simulink model "SystemControl"  (R2019b)
settings: Solver=VariableStepAuto  StartTime=0.0  StopTime=T_sim  RelTol=1e-3
values from neighbouring files (symbols this model uses):
  d_tank = 0.07    [FullSystem.m]    (also in SystemControl_script.m)
  k_m_t = 23.8e-3    (= 0.0238)    [FullSystem.m]    (also in SystemControl_script.m)
  R_load = 1e3    (= 1000)    [FullSystem.m]    (also in SystemControl_script.m)
  T_sim = 5    [FullSystem.m]    (also in SystemControl_script.m = 10; model_1.m = 24)
undefined symbols (not defined in the file or in its folder): columns, DiscIntNeverNeededParam, I_LED_max, V_electrolyzer, V_network
libraries: simulink x5
settings Model: Creator=thequ  LastModifiedBy=thequ

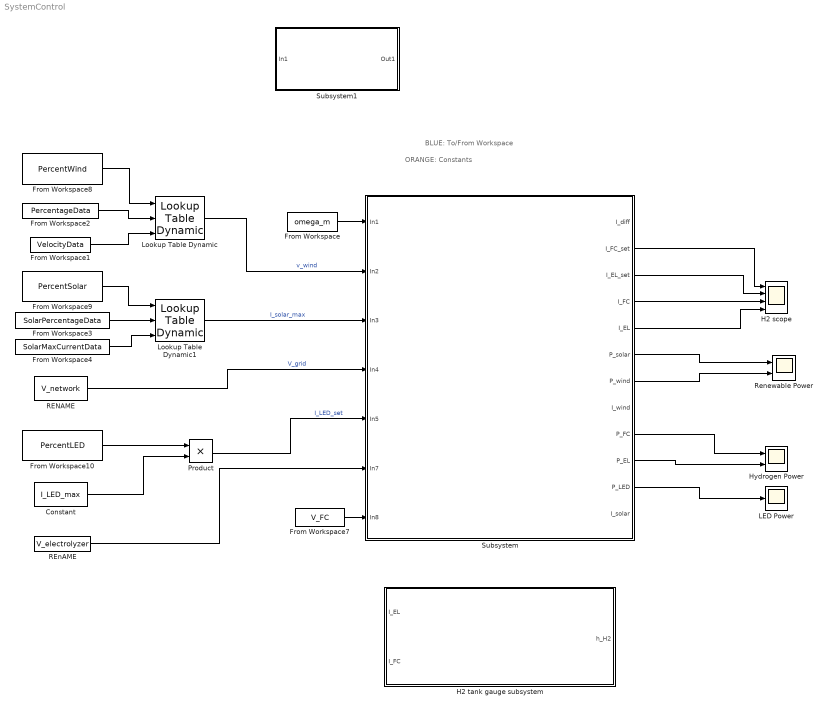
== system SystemControl ==
  note: ORANGE: Constants
  note: BLUE: To/From Workspace
  Constant : Constant  Value=I_LED_max
  From Workspace : FromWorkspace  VariableName=omega_m  SampleTime=T_sim/(columns-1)  Interpolate=off  OutputAfterFinalValue=Holding final value
  From Workspace1 : FromWorkspace  VariableName=VelocityData  SampleTime=0
  From Workspace10 : FromWorkspace  VariableName=PercentLED  SampleTime=0
  From Workspace2 : FromWorkspace  VariableName=PercentageData  SampleTime=0
  From Workspace3 : FromWorkspace  VariableName=SolarPercentageData  SampleTime=0
  From Workspace4 : FromWorkspace  VariableName=SolarMaxCurrentData  SampleTime=0
  From Workspace7 : FromWorkspace  VariableName=V_FC  SampleTime=T_sim/(columns-1)  Interpolate=off  OutputAfterFinalValue=Holding final value
  From Workspace8 : FromWorkspace  VariableName=PercentWind  SampleTime=0
  From Workspace9 : FromWorkspace  VariableName=PercentSolar  SampleTime=0
  H2 scope : Scope  NumInputPorts=4
  H2 tank gauge subsystem : Subsystem
  Hydrogen Power : Scope  NumInputPorts=2
  LED Power : Scope
  Lookup Table Dynamic : simulink/Lookup Tables/Lookup Table Dynamic  LookUpMeth=Interpolation-Use End Values  OutDataType=fixdt('double')  OutScaling=[]  OutputDataTypeScalingMode=Specify via dialog  OutDataTypeStr=double  DoSatur=off
      settings: SourceProductName=Simulink
  Lookup Table Dynamic1 : simulink/Lookup Tables/Lookup Table Dynamic  LookUpMeth=Interpolation-Use End Values  OutDataType=fixdt('double')  OutScaling=[]  OutputDataTypeScalingMode=Specify via dialog  OutDataTypeStr=double  DoSatur=off
      settings: SourceProductName=Simulink
  Product : Product
  RENAME : Constant  Value=V_network
  REnAME : Constant  Value=V_electrolyzer
  Renewable Power : Scope  NumInputPorts=2
  Subsystem : Subsystem
  Subsystem1 : Subsystem
  wires:
  From Workspace/1 -> Subsystem/1(In1)
  Lookup Table Dynamic/1 -> Subsystem/2(In2)  "v_wind"
  Lookup Table Dynamic1/1 -> Subsystem/3(In3)  "I_solar_max"
  RENAME/1 -> Subsystem/4(In4)  "V_grid"
  Product/1 -> Subsystem/5(In5)  "I_LED_set"
  REnAME/1 -> Subsystem/6(In7)
  From Workspace7/1 -> Subsystem/7(In8)
  Subsystem/2(I_FC_set) -> H2 scope/1
  Subsystem/3(I_EL_set) -> H2 scope/2
  Subsystem/6(P_solar) -> Renewable Power/1
  Subsystem/7(P_wind) -> Renewable Power/2
  Subsystem/9(P_FC) -> Hydrogen Power/1
  Subsystem/10(P_EL) -> Hydrogen Power/2
  Subsystem/11(P_LED) -> LED Power/1
  Constant/1 -> Product/2
  From Workspace10/1 -> Product/1
  From Workspace9/1 -> Lookup Table Dynamic1/1
  Subsystem/4(I_FC) -> H2 scope/3
  Subsystem/5(I_EL) -> H2 scope/4
  From Workspace1/1 -> Lookup Table Dynamic/3
  From Workspace2/1 -> Lookup Table Dynamic/2
  From Workspace8/1 -> Lookup Table Dynamic/1
  From Workspace3/1 -> Lookup Table Dynamic1/2
  From Workspace4/1 -> Lookup Table Dynamic1/3

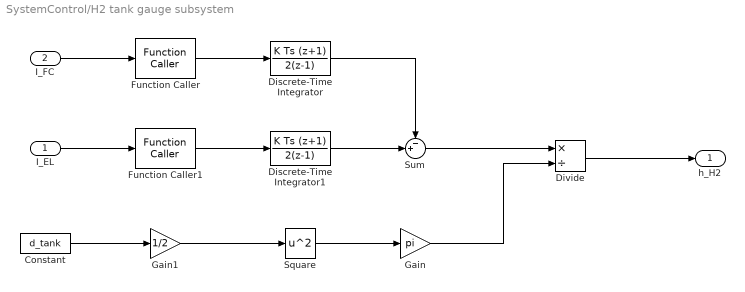
== system SystemControl/H2 tank gauge subsystem ==
  I_EL : Inport
  I_FC : Inport  Port=2
  Constant : Constant  Value=d_tank
  Discrete-Time Integrator : DiscreteIntegrator  IntegratorMethod=Integration: Trapezoidal  SampleTime=-1  ICPrevOutput=DiscIntNeverNeededParam  ICPrevScaledInput=DiscIntNeverNeededParam
  Discrete-Time Integrator1 : DiscreteIntegrator  IntegratorMethod=Integration: Trapezoidal  SampleTime=-1  ICPrevOutput=DiscIntNeverNeededParam  ICPrevScaledInput=DiscIntNeverNeededParam
  Divide : Product  Inputs=*/
  Function Caller : FunctionCaller  FunctionPrototype=y = f(u)  InputArgumentSpecifications=<Enter example>  OutputArgumentSpecifications=<Enter example>
  Function Caller1 : FunctionCaller  FunctionPrototype=y = f(u)  InputArgumentSpecifications=<Enter example>  OutputArgumentSpecifications=<Enter example>
  Gain : Gain  Gain=pi
  Gain1 : Gain  Gain=1/2
  Square : Math  Operator=square  SignedPower=off  SaturateOnIntegerOverflow=on
  Sum : Sum  Inputs=-+|
  h_H2 : Outport
  wires:
  I_FC/1 -> Function Caller/1
  I_EL/1 -> Function Caller1/1
  Function Caller/1 -> Discrete-Time Integrator/1
  Function Caller1/1 -> Discrete-Time Integrator1/1
  Constant/1 -> Gain1/1
  Discrete-Time Integrator1/1 -> Sum/2
  Discrete-Time Integrator/1 -> Sum/1
  Gain1/1 -> Square/1
  Square/1 -> Gain/1
  Gain/1 -> Divide/2
  Sum/1 -> Divide/1
  Divide/1 -> h_H2/1

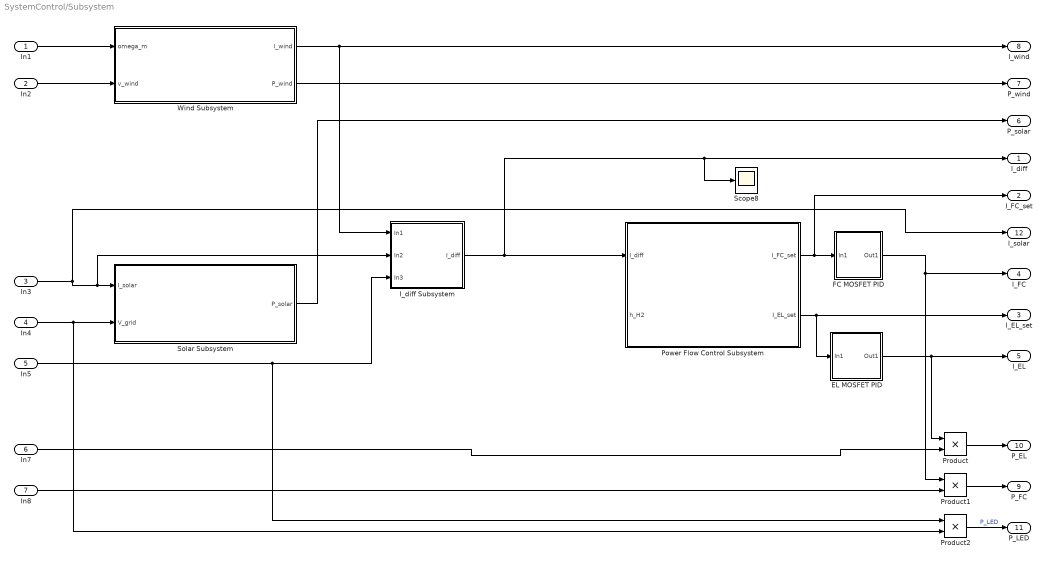
== system SystemControl/Subsystem ==
  In1 : Inport
  In2 : Inport  Port=2
  In3 : Inport  Port=3
  In4 : Inport  Port=4
  In5 : Inport  Port=5
  In7 : Inport  Port=6
  In8 : Inport  Port=7
  EL MOSFET PID : Subsystem
  FC MOSFET PID : Subsystem
  I_diff Subsystem : Subsystem
  Power Flow Control Subsystem : Subsystem
  Product : Product
  Product1 : Product
  Product2 : Product
  Scope8 : Scope
  Solar Subsystem : Subsystem
  "Wind Subsystem " : Subsystem
  I_diff : Outport
  I_FC_set : Outport  Port=2
  I_EL_set : Outport  Port=3
  I_FC : Outport  Port=4
  I_EL : Outport  Port=5
  P_solar : Outport  Port=6
  P_wind : Outport  Port=7
  I_wind : Outport  Port=8
  P_FC : Outport  Port=9
  P_EL : Outport  Port=10
  P_LED : Outport  Port=11
  I_solar : Outport  Port=12
  wires:
  Product2/1 -> P_LED/1  "P_LED"
  I_diff Subsystem/1(I_diff) -> I_diff/1, Scope8/1, Power Flow Control Subsystem/1(I_diff)
  In4/1 -> Product2/2, Solar Subsystem/2(V_grid)
  Power Flow Control Subsystem/2(I_EL_set) -> I_EL_set/1, EL MOSFET PID/1(In1)
  Power Flow Control Subsystem/1(I_FC_set) -> I_FC_set/1, FC MOSFET PID/1(In1)
  EL MOSFET PID/1(Out1) -> I_EL/1, Product/1
  FC MOSFET PID/1(Out1) -> I_FC/1, Product1/1
  In3/1 -> I_diff Subsystem/2(In2), Solar Subsystem/1(I_solar), I_solar/1
  "Wind Subsystem "/2("P_wind ") -> P_wind/1
  "Wind Subsystem "/1("I_wind ") -> I_diff Subsystem/1(In1), I_wind/1
  In5/1 -> Product2/1, I_diff Subsystem/3(In3)
  Product/1 -> P_EL/1
  In1/1 -> "Wind Subsystem "/1(omega_m)
  Product1/1 -> P_FC/1
  Solar Subsystem/1(P_solar) -> P_solar/1
  In2/1 -> "Wind Subsystem "/2("v_wind ")
  In8/1 -> Product1/2
  In7/1 -> Product/2

== system SystemControl/Subsystem1 ==
  In1 : Inport
  Out1 : Outport
  wires:
  In1/1 -> Out1/1

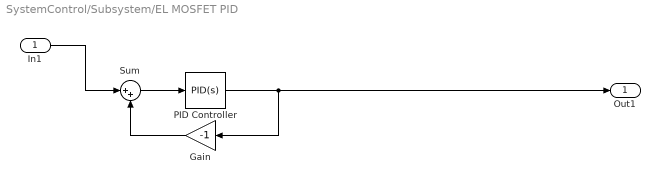
== system SystemControl/Subsystem/EL MOSFET PID ==
  In1 : Inport
  Gain : Gain  Gain=-1
  PID Controller : simulink/Continuous/PID Controller  Controller=PID  Form=Parallel  TimeDomain=Continuous-time  SampleTime=-1  IntegratorMethod=Forward Euler  FilterMethod=Forward Euler  ControllerParametersSource=internal  P=6  I=1  D=0  UseFilter=on  N=100  TunerSelectOption=Transfer Function Based (PID Tuner App)  InitialConditionSource=internal  InitialConditionForIntegrator=0  InitialConditionForFilter=0  DifferentiatorICPrevScaledInput=0  ExternalReset=none  TrackingMode=off  Kt=1  LimitOutput=off  UpperSaturationLimit=inf  LowerSaturationLimit=-inf  LinearizeAsGain=on  AntiWindupMode=none  Kb=1  POutMin=[]  POutMax=[]  IOutMin=[]  IOutMax=[]  DOutMin=[]  DOutMax=[]  NOutMin=[]  NOutMax=[]  SumOutMin=[]  SumOutMax=[]  SaturationOutMin=[]  SaturationOutMax=[]  PParamMin=[]  PParamMax=[]  IParamMin=[]  IParamMax=[]  DParamMin=[]  DParamMax=[]  NParamMin=[]  NParamMax=[]  KbParamMin=[]  KbParamMax=[]  KtParamMin=[]  KtParamMax=[]  KbOutMin=[]  KbOutMax=[]  KtOutMin=[]  KtOutMax=[]  IntegratorOutMin=[]  IntegratorOutMax=[]  FilterOutMin=[]  FilterOutMax=[]  SumI1OutMin=[]  SumI1OutMax=[]  SumI2OutMin=[]  SumI2OutMax=[]  SumI3OutMin=[]  SumI3OutMax=[]  SumI4OutMin=[]  SumI4OutMax=[]  SumDOutMin=[]  SumDOutMax=[]  DifferentiatorOutMin=[]  DifferentiatorOutMax=[]  FilterDiffOutCoefMin=[]  FilterDiffOutCoefMax=[]  ReciprocalOutMin=[]  ReciprocalOutMax=[]  SumDenOutMin=[]  SumDenOutMax=[]  SumNumOutMin=[]  SumNumOutMax=[]  DivideOutMin=[]  DivideOutMax=[]  IntegratorContinuousStateAttributes=''  IntegratorStateMustResolveToSignalObject=off  IntegratorRTWStateStorageClass=Auto  FilterContinuousStateAttributes=''  FilterStateMustResolveToSignalObject=off  FilterRTWStateStorageClass=Auto  ParallelPVariant=InternalParameters  IdealPVariant=Disabled  IVariant=InternalParameters  DVariant=InternalParameters  IntegratorVariant=Continuous  SatVariant=Disabled  AWVariant=Passthrough  PCopyVariant=Disabled  TRVariant=Disabled  FdbkBlocksVariant=Forward  IdealPFdbkVariant=Disabled  SatFdbkVariant=Disabled  DerivativeFilterVariant=ContFilter  NVariant=InternalParameters  NCopyVariant=Disabled  FilterICVariant=InternalICsFilter  IntegratorICVariant=InternalICs  ExternalResetVariant=Disabled  TRSumVariant=Passthrough  SumFdbkVariant=Disabled  SumVariant=Sum_PID
  Sum : Sum  Inputs=|++
  Out1 : Outport
  wires:
  Sum/1 -> PID Controller/1
  Gain/1 -> Sum/2
  In1/1 -> Sum/1
  PID Controller/1 -> Out1/1, Gain/1

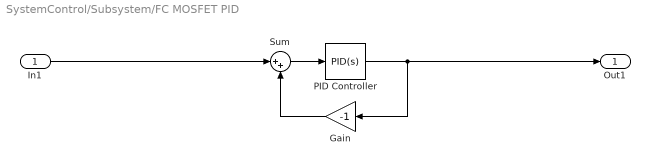
== system SystemControl/Subsystem/FC MOSFET PID ==
  In1 : Inport
  Gain : Gain  Gain=-1
  PID Controller : simulink/Continuous/PID Controller  Controller=PID  Form=Parallel  TimeDomain=Continuous-time  SampleTime=-1  IntegratorMethod=Forward Euler  FilterMethod=Forward Euler  ControllerParametersSource=internal  P=1  I=0  D=0  UseFilter=on  N=100  TunerSelectOption=Transfer Function Based (PID Tuner App)  InitialConditionSource=internal  InitialConditionForIntegrator=0  InitialConditionForFilter=0  DifferentiatorICPrevScaledInput=0  ExternalReset=none  TrackingMode=off  Kt=1  LimitOutput=off  UpperSaturationLimit=inf  LowerSaturationLimit=-inf  LinearizeAsGain=on  AntiWindupMode=none  Kb=1  POutMin=[]  POutMax=[]  IOutMin=[]  IOutMax=[]  DOutMin=[]  DOutMax=[]  NOutMin=[]  NOutMax=[]  SumOutMin=[]  SumOutMax=[]  SaturationOutMin=[]  SaturationOutMax=[]  PParamMin=[]  PParamMax=[]  IParamMin=[]  IParamMax=[]  DParamMin=[]  DParamMax=[]  NParamMin=[]  NParamMax=[]  KbParamMin=[]  KbParamMax=[]  KtParamMin=[]  KtParamMax=[]  KbOutMin=[]  KbOutMax=[]  KtOutMin=[]  KtOutMax=[]  IntegratorOutMin=[]  IntegratorOutMax=[]  FilterOutMin=[]  FilterOutMax=[]  SumI1OutMin=[]  SumI1OutMax=[]  SumI2OutMin=[]  SumI2OutMax=[]  SumI3OutMin=[]  SumI3OutMax=[]  SumI4OutMin=[]  SumI4OutMax=[]  SumDOutMin=[]  SumDOutMax=[]  DifferentiatorOutMin=[]  DifferentiatorOutMax=[]  FilterDiffOutCoefMin=[]  FilterDiffOutCoefMax=[]  ReciprocalOutMin=[]  ReciprocalOutMax=[]  SumDenOutMin=[]  SumDenOutMax=[]  SumNumOutMin=[]  SumNumOutMax=[]  DivideOutMin=[]  DivideOutMax=[]  IntegratorContinuousStateAttributes=''  IntegratorStateMustResolveToSignalObject=off  IntegratorRTWStateStorageClass=Auto  FilterContinuousStateAttributes=''  FilterStateMustResolveToSignalObject=off  FilterRTWStateStorageClass=Auto  ParallelPVariant=InternalParameters  IdealPVariant=Disabled  IVariant=InternalParameters  DVariant=InternalParameters  IntegratorVariant=Continuous  SatVariant=Disabled  AWVariant=Passthrough  PCopyVariant=Disabled  TRVariant=Disabled  FdbkBlocksVariant=Forward  IdealPFdbkVariant=Disabled  SatFdbkVariant=Disabled  DerivativeFilterVariant=ContFilter  NVariant=InternalParameters  NCopyVariant=Disabled  FilterICVariant=InternalICsFilter  IntegratorICVariant=InternalICs  ExternalResetVariant=Disabled  TRSumVariant=Passthrough  SumFdbkVariant=Disabled  SumVariant=Sum_PID
  Sum : Sum  Inputs=|++
  Out1 : Outport
  wires:
  PID Controller/1 -> Out1/1, Gain/1
  Sum/1 -> PID Controller/1
  Gain/1 -> Sum/2
  In1/1 -> Sum/1

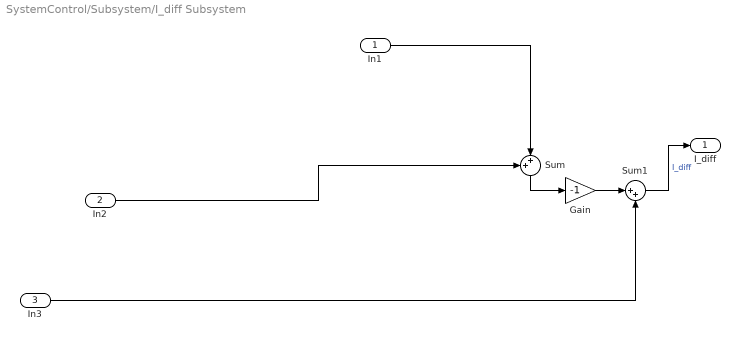
== system SystemControl/Subsystem/I_diff Subsystem ==
  In1 : Inport
  In2 : Inport  Port=2
  In3 : Inport  Port=3
  Gain : Gain  Gain=-1
  Sum : Sum  Inputs=++|
  Sum1 : Sum  Inputs=|++
  I_diff : Outport
  wires:
  Sum1/1 -> I_diff/1  "I_diff"
  Gain/1 -> Sum1/1
  Sum/1 -> Gain/1
  In1/1 -> Sum/2
  In3/1 -> Sum1/2
  In2/1 -> Sum/1

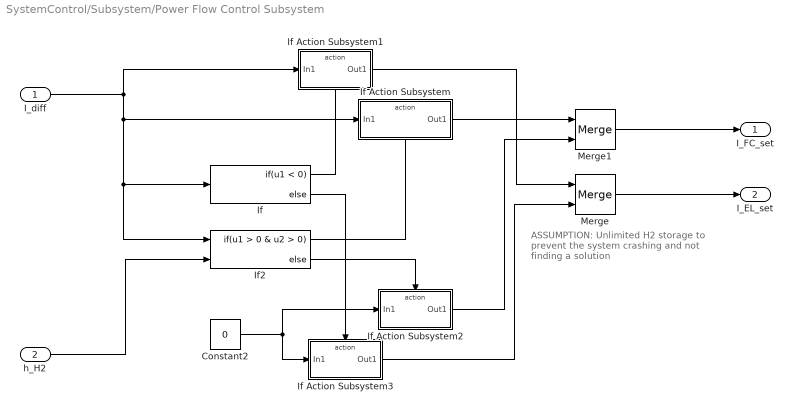
== system SystemControl/Subsystem/Power Flow Control Subsystem ==
  note: ASSUMPTION: Unlimited H2 storage to
      | prevent the system crashing and not
      | finding a solution
  I_diff : Inport
  h_H2 : Inport  Port=2
  Constant2 : Constant  Value=0
  If : If  IfExpression=u1 < 0
  If Action Subsystem : Subsystem  TreatAsAtomicUnit=on
  If Action Subsystem1 : Subsystem  TreatAsAtomicUnit=on
  If Action Subsystem2 : Subsystem  TreatAsAtomicUnit=on
  If Action Subsystem3 : Subsystem  TreatAsAtomicUnit=on
  If2 : If  NumInputs=2  IfExpression=u1 > 0 & u2 > 0
  Merge : Merge
  Merge1 : Merge
  I_FC_set : Outport
  I_EL_set : Outport  Port=2
  wires:
  Merge/1 -> I_EL_set/1
  If Action Subsystem2/1(Out1) -> Merge1/2
  Merge1/1 -> I_FC_set/1
  I_diff/1 -> If/1, If2/1, If Action Subsystem/1(In1), If Action Subsystem1/1(In1)
  Constant2/1 -> If Action Subsystem3/1(In1), If Action Subsystem2/1(In1)
  If Action Subsystem/1(Out1) -> Merge1/1
  If Action Subsystem3/1(Out1) -> Merge/2
  h_H2/1 -> If2/2
  If2/1 -> If Action Subsystem/Action
  If2/2 -> If Action Subsystem2/Action
  If/2 -> If Action Subsystem3/Action
  If/1 -> If Action Subsystem1/Action
  If Action Subsystem1/1(Out1) -> Merge/1

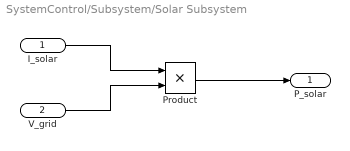
== system SystemControl/Subsystem/Solar Subsystem ==
  I_solar : Inport
  V_grid : Inport  Port=2
  Product : Product
  P_solar : Outport
  wires:
  V_grid/1 -> Product/2
  I_solar/1 -> Product/1
  Product/1 -> P_solar/1

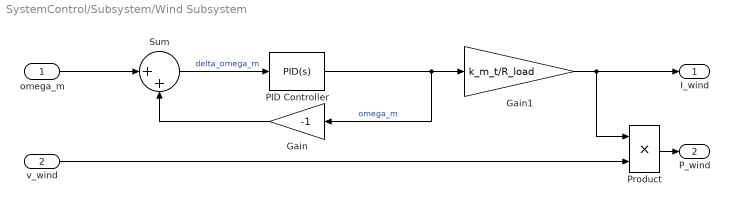
== system SystemControl/Subsystem/Wind Subsystem  ==
  omega_m : Inport
  "v_wind " : Inport  Port=2
  Gain : Gain  Gain=-1
  Gain1 : Gain  Gain=k_m_t/R_load
  PID Controller : simulink/Continuous/PID Controller  Controller=PID  Form=Parallel  TimeDomain=Continuous-time  SampleTime=-1  IntegratorMethod=Forward Euler  FilterMethod=Forward Euler  ControllerParametersSource=internal  P=1  I=0  D=0  UseFilter=on  N=100  TunerSelectOption=Transfer Function Based (PID Tuner App)  InitialConditionSource=internal  InitialConditionForIntegrator=0  InitialConditionForFilter=0  DifferentiatorICPrevScaledInput=0  ExternalReset=none  TrackingMode=off  Kt=1  LimitOutput=off  UpperSaturationLimit=inf  LowerSaturationLimit=-inf  LinearizeAsGain=on  AntiWindupMode=none  Kb=1  POutMin=[]  POutMax=[]  IOutMin=[]  IOutMax=[]  DOutMin=[]  DOutMax=[]  NOutMin=[]  NOutMax=[]  SumOutMin=[]  SumOutMax=[]  SaturationOutMin=[]  SaturationOutMax=[]  PParamMin=[]  PParamMax=[]  IParamMin=[]  IParamMax=[]  DParamMin=[]  DParamMax=[]  NParamMin=[]  NParamMax=[]  KbParamMin=[]  KbParamMax=[]  KtParamMin=[]  KtParamMax=[]  KbOutMin=[]  KbOutMax=[]  KtOutMin=[]  KtOutMax=[]  IntegratorOutMin=[]  IntegratorOutMax=[]  FilterOutMin=[]  FilterOutMax=[]  SumI1OutMin=[]  SumI1OutMax=[]  SumI2OutMin=[]  SumI2OutMax=[]  SumI3OutMin=[]  SumI3OutMax=[]  SumI4OutMin=[]  SumI4OutMax=[]  SumDOutMin=[]  SumDOutMax=[]  DifferentiatorOutMin=[]  DifferentiatorOutMax=[]  FilterDiffOutCoefMin=[]  FilterDiffOutCoefMax=[]  ReciprocalOutMin=[]  ReciprocalOutMax=[]  SumDenOutMin=[]  SumDenOutMax=[]  SumNumOutMin=[]  SumNumOutMax=[]  DivideOutMin=[]  DivideOutMax=[]  IntegratorContinuousStateAttributes=''  IntegratorStateMustResolveToSignalObject=off  IntegratorRTWStateStorageClass=Auto  FilterContinuousStateAttributes=''  FilterStateMustResolveToSignalObject=off  FilterRTWStateStorageClass=Auto  ParallelPVariant=InternalParameters  IdealPVariant=Disabled  IVariant=InternalParameters  DVariant=InternalParameters  IntegratorVariant=Continuous  SatVariant=Disabled  AWVariant=Passthrough  PCopyVariant=Disabled  TRVariant=Disabled  FdbkBlocksVariant=Forward  IdealPFdbkVariant=Disabled  SatFdbkVariant=Disabled  DerivativeFilterVariant=ContFilter  NVariant=InternalParameters  NCopyVariant=Disabled  FilterICVariant=InternalICsFilter  IntegratorICVariant=InternalICs  ExternalResetVariant=Disabled  TRSumVariant=Passthrough  SumFdbkVariant=Disabled  SumVariant=Sum_PID
  Product : Product
  Sum : Sum  Inputs=|++
  "I_wind " : Outport
  "P_wind " : Outport  Port=2
  wires:
  Gain/1 -> Sum/2
  Sum/1 -> PID Controller/1  "delta_omega_m"
  omega_m/1 -> Sum/1
  PID Controller/1 -> Gain1/1, Gain/1  "omega_m"
  Gain1/1 -> "I_wind "/1, Product/1
  Product/1 -> "P_wind "/1
  "v_wind "/1 -> Product/2

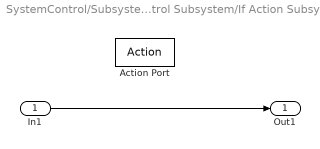
== system SystemControl/Subsystem/Power Flow Control Subsystem/If Action Subsystem ==
  In1 : Inport
  Action Port : ActionPort  ActionPortLabel=if(u1 > 0 & u2 > 0)
  Out1 : Outport
  wires:
  In1/1 -> Out1/1

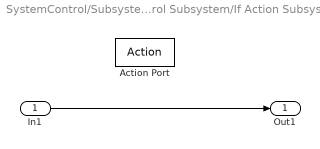
== system SystemControl/Subsystem/Power Flow Control Subsystem/If Action Subsystem1 ==
  In1 : Inport
  Action Port : ActionPort  ActionPortLabel=if(u1 < 0)
  Out1 : Outport
  wires:
  In1/1 -> Out1/1

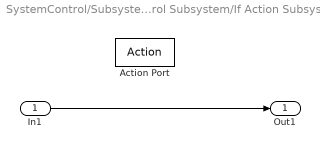
== system SystemControl/Subsystem/Power Flow Control Subsystem/If Action Subsystem2 ==
  In1 : Inport
  Action Port : ActionPort  ActionPortLabel=else
  Out1 : Outport
  wires:
  In1/1 -> Out1/1

== system SystemControl/Subsystem/Power Flow Control Subsystem/If Action Subsystem3 ==
  In1 : Inport
  Action Port : ActionPort  ActionPortLabel=else
  Out1 : Outport
  wires:
  In1/1 -> Out1/1
